simulink model "TCMSSystem"  (R2019b)
settings: configuration reference "ConfigSet_TCMSSystem_Reference" (kept outside this file)
model workspace (MAT data in the model file):
  Prm_TCMSSystem : Simulink.Parameter (value not decoded)
  SampleTime = 0.05
symbols that are objects in the model workspace (value not decoded): Prm_TCMSSystem
undefined symbols (not defined in the file): ADDIntervention, AK1Status, AK2Status, AKContactorStatus, AllDoorsClosed, AllLeftDoorsClosed, AllRightDoorsClosed, APS1Fault, APS1Isolated, APS1OutputVoltage, APS1Status, APS2Fault, APS2Isolated, APS2OutputVoltage, APS2Status, APSKAKContactor, ASCOEnd1, ASCOEnd2, ATBMode, ATCBypassMode, ATCStatusNotOK, ATOMode, ATPLowSpeedCutoutStatus, ATPMode, AuxCompressor, BatteryCurrent, BatteryIsolationContactor, BatteryTemperature, BatteryVoltage, BCG1Fault, BCG1Isolated, BCG1IsolationFailed, BCG1OutputCurrent, BCG1Status, BCG2Fault, BCG2Isolated, BCG2OutputCurrent, BCG2Status, BCGOutputVoltage, BECU1AxleLockedWheelSet1, BECU2AxleLockedWheelSet2, BECUFaulty, BECUMajorFault, BECUMinorFault, BECUStatus, BIC1Inside, BIC1Outside, BIC2Inside, BIC2Outside, Bogie, Bogie1WSPStatus, Bogie2WSPStatus, BogieFaulty, BogieIsolationStatus, BogieSupportedMass, BrakeCylinderPressureGauge, BrakeLoopCBTripped, BrakeLoopOpenTL, BrakeTrainLineStatus, BrakingDemand ... (+215)
libraries: TimersLib x257, simulink x137, LatchesLib x42, VectorOperationsLib x15, TestBenchLib x12, MathOperationsLib x2, FiltersLib x1
(part 15 of 16)

== system TCMSSystem/TCMSSystemPerVehicle/EnabledTCMSVehicle/OutputsPacking/TCMSDisplayOutputs/TCMSMessageEvents/New46EventsMessage/Associated TCMS Fault ID42 ==
  State : Inport
  Bus Creator1 : BusCreator  Inputs=2  OutDataTypeStr=Bus: BD_TCMSSystem_Out_Vehicle_Display_Message  NonVirtualBus=on
  Constant : Constant  Value=MessageID
  Data Type Conversion : DataTypeConversion
  Message : Outport  VectorParamsAs1DForOutWhenUnconnected=off
  wires:
  Data Type Conversion/1 -> Bus Creator1/2  "MessageStatus"
  Constant/1 -> Bus Creator1/1  "MessageID"
  State/1 -> Data Type Conversion/1
  Bus Creator1/1 -> Message/1

== system TCMSSystem/TCMSSystemPerVehicle/EnabledTCMSVehicle/OutputsPacking/TCMSDisplayOutputs/TCMSMessageEvents/New46EventsMessage/Associated TCMS Fault ID43 ==
  State : Inport
  Bus Creator1 : BusCreator  Inputs=2  OutDataTypeStr=Bus: BD_TCMSSystem_Out_Vehicle_Display_Message  NonVirtualBus=on
  Constant : Constant  Value=MessageID
  Data Type Conversion : DataTypeConversion
  Message : Outport  VectorParamsAs1DForOutWhenUnconnected=off
  wires:
  Bus Creator1/1 -> Message/1
  State/1 -> Data Type Conversion/1
  Constant/1 -> Bus Creator1/1  "MessageID"
  Data Type Conversion/1 -> Bus Creator1/2  "MessageStatus"

== system TCMSSystem/TCMSSystemPerVehicle/EnabledTCMSVehicle/OutputsPacking/TCMSDisplayOutputs/TCMSMessageEvents/New46EventsMessage/Associated TCMS Fault ID44 ==
  State : Inport
  Bus Creator1 : BusCreator  Inputs=2  OutDataTypeStr=Bus: BD_TCMSSystem_Out_Vehicle_Display_Message  NonVirtualBus=on
  Constant : Constant  Value=MessageID
  Data Type Conversion : DataTypeConversion
  Message : Outport  VectorParamsAs1DForOutWhenUnconnected=off
  wires:
  Data Type Conversion/1 -> Bus Creator1/2  "MessageStatus"
  Constant/1 -> Bus Creator1/1  "MessageID"
  State/1 -> Data Type Conversion/1
  Bus Creator1/1 -> Message/1

== system TCMSSystem/TCMSSystemPerVehicle/EnabledTCMSVehicle/OutputsPacking/TCMSDisplayOutputs/TCMSMessageEvents/New46EventsMessage/Associated TCMS Fault ID45 ==
  State : Inport
  Bus Creator1 : BusCreator  Inputs=2  OutDataTypeStr=Bus: BD_TCMSSystem_Out_Vehicle_Display_Message  NonVirtualBus=on
  Constant : Constant  Value=MessageID
  Data Type Conversion : DataTypeConversion
  Message : Outport  VectorParamsAs1DForOutWhenUnconnected=off
  wires:
  Data Type Conversion/1 -> Bus Creator1/2  "MessageStatus"
  Constant/1 -> Bus Creator1/1  "MessageID"
  State/1 -> Data Type Conversion/1
  Bus Creator1/1 -> Message/1

== system TCMSSystem/TCMSSystemPerVehicle/EnabledTCMSVehicle/OutputsPacking/TCMSDisplayOutputs/TCMSMessageEvents/New46EventsMessage/Associated TCMS Fault ID46 ==
  State : Inport
  Bus Creator1 : BusCreator  Inputs=2  OutDataTypeStr=Bus: BD_TCMSSystem_Out_Vehicle_Display_Message  NonVirtualBus=on
  Constant : Constant  Value=MessageID
  Data Type Conversion : DataTypeConversion
  Message : Outport  VectorParamsAs1DForOutWhenUnconnected=off
  wires:
  Bus Creator1/1 -> Message/1
  State/1 -> Data Type Conversion/1
  Constant/1 -> Bus Creator1/1  "MessageID"
  Data Type Conversion/1 -> Bus Creator1/2  "MessageStatus"

== system TCMSSystem/TCMSSystemPerVehicle/EnabledTCMSVehicle/OutputsPacking/TCMSDisplayOutputs/TCMSMessageEvents/New46EventsMessage/Associated TCMS Fault ID47 ==
  State : Inport
  Bus Creator1 : BusCreator  Inputs=2  OutDataTypeStr=Bus: BD_TCMSSystem_Out_Vehicle_Display_Message  NonVirtualBus=on
  Constant : Constant  Value=MessageID
  Data Type Conversion : DataTypeConversion
  Message : Outport  VectorParamsAs1DForOutWhenUnconnected=off
  wires:
  Data Type Conversion/1 -> Bus Creator1/2  "MessageStatus"
  Constant/1 -> Bus Creator1/1  "MessageID"
  State/1 -> Data Type Conversion/1
  Bus Creator1/1 -> Message/1

== system TCMSSystem/TCMSSystemPerVehicle/EnabledTCMSVehicle/OutputsPacking/TCMSDisplayOutputs/TCMSMessageEvents/New46EventsMessage/Associated TCMS Fault ID48 ==
  State : Inport
  Bus Creator1 : BusCreator  Inputs=2  OutDataTypeStr=Bus: BD_TCMSSystem_Out_Vehicle_Display_Message  NonVirtualBus=on
  Constant : Constant  Value=MessageID
  Data Type Conversion : DataTypeConversion
  Message : Outport  VectorParamsAs1DForOutWhenUnconnected=off
  wires:
  Bus Creator1/1 -> Message/1
  State/1 -> Data Type Conversion/1
  Constant/1 -> Bus Creator1/1  "MessageID"
  Data Type Conversion/1 -> Bus Creator1/2  "MessageStatus"

== system TCMSSystem/TCMSSystemPerVehicle/EnabledTCMSVehicle/OutputsPacking/TCMSDisplayOutputs/TCMSMessageEvents/New46EventsMessage/Associated TCMS Fault ID50 ==
  State : Inport
  Bus Creator1 : BusCreator  Inputs=2  OutDataTypeStr=Bus: BD_TCMSSystem_Out_Vehicle_Display_Message  NonVirtualBus=on
  Constant : Constant  Value=MessageID
  Data Type Conversion : DataTypeConversion
  Message : Outport  VectorParamsAs1DForOutWhenUnconnected=off
  wires:
  Bus Creator1/1 -> Message/1
  State/1 -> Data Type Conversion/1
  Constant/1 -> Bus Creator1/1  "MessageID"
  Data Type Conversion/1 -> Bus Creator1/2  "MessageStatus"

== system TCMSSystem/TCMSSystemPerVehicle/EnabledTCMSVehicle/OutputsPacking/TCMSDisplayOutputs/TCMSMessageEvents/New46EventsMessage/Associated TCMS Fault ID53 ==
  State : Inport
  Bus Creator1 : BusCreator  Inputs=2  OutDataTypeStr=Bus: BD_TCMSSystem_Out_Vehicle_Display_Message  NonVirtualBus=on
  Constant : Constant  Value=MessageID
  Data Type Conversion : DataTypeConversion
  Message : Outport  VectorParamsAs1DForOutWhenUnconnected=off
  wires:
  Bus Creator1/1 -> Message/1
  State/1 -> Data Type Conversion/1
  Constant/1 -> Bus Creator1/1  "MessageID"
  Data Type Conversion/1 -> Bus Creator1/2  "MessageStatus"

== system TCMSSystem/TCMSSystemPerVehicle/EnabledTCMSVehicle/OutputsPacking/TCMSDisplayOutputs/TCMSMessageEvents/New46EventsMessage/Associated TCMS Fault ID54 ==
  State : Inport
  Bus Creator1 : BusCreator  Inputs=2  OutDataTypeStr=Bus: BD_TCMSSystem_Out_Vehicle_Display_Message  NonVirtualBus=on
  Constant : Constant  Value=MessageID
  Data Type Conversion : DataTypeConversion
  Message : Outport  VectorParamsAs1DForOutWhenUnconnected=off
  wires:
  Data Type Conversion/1 -> Bus Creator1/2  "MessageStatus"
  Constant/1 -> Bus Creator1/1  "MessageID"
  State/1 -> Data Type Conversion/1
  Bus Creator1/1 -> Message/1

== system TCMSSystem/TCMSSystemPerVehicle/EnabledTCMSVehicle/OutputsPacking/TCMSDisplayOutputs/TCMSMessageEvents/New46EventsMessage/Associated TCMS Fault ID55 ==
  State : Inport
  Bus Creator1 : BusCreator  Inputs=2  OutDataTypeStr=Bus: BD_TCMSSystem_Out_Vehicle_Display_Message  NonVirtualBus=on
  Constant : Constant  Value=MessageID
  Data Type Conversion : DataTypeConversion
  Message : Outport  VectorParamsAs1DForOutWhenUnconnected=off
  wires:
  Bus Creator1/1 -> Message/1
  State/1 -> Data Type Conversion/1
  Constant/1 -> Bus Creator1/1  "MessageID"
  Data Type Conversion/1 -> Bus Creator1/2  "MessageStatus"

== system TCMSSystem/TCMSSystemPerVehicle/EnabledTCMSVehicle/OutputsPacking/TCMSDisplayOutputs/TCMSMessageEvents/New46EventsMessage/Associated TCMS Fault ID56 ==
  State : Inport
  Bus Creator1 : BusCreator  Inputs=2  OutDataTypeStr=Bus: BD_TCMSSystem_Out_Vehicle_Display_Message  NonVirtualBus=on
  Constant : Constant  Value=MessageID
  Data Type Conversion : DataTypeConversion
  Message : Outport  VectorParamsAs1DForOutWhenUnconnected=off
  wires:
  Data Type Conversion/1 -> Bus Creator1/2  "MessageStatus"
  Constant/1 -> Bus Creator1/1  "MessageID"
  State/1 -> Data Type Conversion/1
  Bus Creator1/1 -> Message/1

== system TCMSSystem/TCMSSystemPerVehicle/EnabledTCMSVehicle/OutputsPacking/TCMSDisplayOutputs/TCMSMessageEvents/New46EventsMessage/Associated TCMS Fault ID57 ==
  State : Inport
  Bus Creator1 : BusCreator  Inputs=2  OutDataTypeStr=Bus: BD_TCMSSystem_Out_Vehicle_Display_Message  NonVirtualBus=on
  Constant : Constant  Value=MessageID
  Data Type Conversion : DataTypeConversion
  Message : Outport  VectorParamsAs1DForOutWhenUnconnected=off
  wires:
  Bus Creator1/1 -> Message/1
  State/1 -> Data Type Conversion/1
  Constant/1 -> Bus Creator1/1  "MessageID"
  Data Type Conversion/1 -> Bus Creator1/2  "MessageStatus"

== system TCMSSystem/TCMSSystemPerVehicle/EnabledTCMSVehicle/OutputsPacking/TCMSDisplayOutputs/TCMSMessageEvents/New46EventsMessage/Associated TCMS Fault ID6 ==
  State : Inport
  Bus Creator1 : BusCreator  Inputs=2  OutDataTypeStr=Bus: BD_TCMSSystem_Out_Vehicle_Display_Message  NonVirtualBus=on
  Constant : Constant  Value=MessageID
  Data Type Conversion : DataTypeConversion
  Message : Outport  VectorParamsAs1DForOutWhenUnconnected=off
  wires:
  Bus Creator1/1 -> Message/1
  State/1 -> Data Type Conversion/1
  Constant/1 -> Bus Creator1/1  "MessageID"
  Data Type Conversion/1 -> Bus Creator1/2  "MessageStatus"

== system TCMSSystem/TCMSSystemPerVehicle/EnabledTCMSVehicle/OutputsPacking/TCMSDisplayOutputs/TCMSMessageEvents/New46EventsMessage/Associated TCMS Fault ID7 ==
  State : Inport
  Bus Creator1 : BusCreator  Inputs=2  OutDataTypeStr=Bus: BD_TCMSSystem_Out_Vehicle_Display_Message  NonVirtualBus=on
  Constant : Constant  Value=MessageID
  Data Type Conversion : DataTypeConversion
  Message : Outport  VectorParamsAs1DForOutWhenUnconnected=off
  wires:
  Data Type Conversion/1 -> Bus Creator1/2  "MessageStatus"
  Constant/1 -> Bus Creator1/1  "MessageID"
  State/1 -> Data Type Conversion/1
  Bus Creator1/1 -> Message/1

== system TCMSSystem/TCMSSystemPerVehicle/EnabledTCMSVehicle/OutputsPacking/TCMSDisplayOutputs/TCMSMessageEvents/New46EventsMessage/Associated TCMS Fault ID8 ==
  State : Inport
  Bus Creator1 : BusCreator  Inputs=2  OutDataTypeStr=Bus: BD_TCMSSystem_Out_Vehicle_Display_Message  NonVirtualBus=on
  Constant : Constant  Value=MessageID
  Data Type Conversion : DataTypeConversion
  Message : Outport  VectorParamsAs1DForOutWhenUnconnected=off
  wires:
  Bus Creator1/1 -> Message/1
  State/1 -> Data Type Conversion/1
  Constant/1 -> Bus Creator1/1  "MessageID"
  Data Type Conversion/1 -> Bus Creator1/2  "MessageStatus"

== system TCMSSystem/TCMSSystemPerVehicle/EnabledTCMSVehicle/OutputsPacking/TCMSDisplayOutputs/TCMSMessageEvents/PantographSystemFaults/Associated TCMS Fault ID24 ==
  State : Inport
  Bus Creator1 : BusCreator  Inputs=2  OutDataTypeStr=Bus: BD_TCMSSystem_Out_Vehicle_Display_Message  NonVirtualBus=on
  Constant : Constant  Value=MessageID
  Data Type Conversion : DataTypeConversion
  Message : Outport  VectorParamsAs1DForOutWhenUnconnected=off
  wires:
  Bus Creator1/1 -> Message/1
  State/1 -> Data Type Conversion/1
  Constant/1 -> Bus Creator1/1  "MessageID"
  Data Type Conversion/1 -> Bus Creator1/2  "MessageStatus"

== system TCMSSystem/TCMSSystemPerVehicle/EnabledTCMSVehicle/OutputsPacking/TCMSDisplayOutputs/TCMSMessageEvents/PantographSystemFaults/Associated TCMS Fault ID25 ==
  State : Inport
  Bus Creator1 : BusCreator  Inputs=2  OutDataTypeStr=Bus: BD_TCMSSystem_Out_Vehicle_Display_Message  NonVirtualBus=on
  Constant : Constant  Value=MessageID
  Data Type Conversion : DataTypeConversion
  Message : Outport  VectorParamsAs1DForOutWhenUnconnected=off
  wires:
  Data Type Conversion/1 -> Bus Creator1/2  "MessageStatus"
  Constant/1 -> Bus Creator1/1  "MessageID"
  State/1 -> Data Type Conversion/1
  Bus Creator1/1 -> Message/1

== system TCMSSystem/TCMSSystemPerVehicle/EnabledTCMSVehicle/OutputsPacking/TCMSDisplayOutputs/TCMSMessageEvents/PantographSystemFaults/Associated TCMS Fault ID26 ==
  State : Inport
  Bus Creator1 : BusCreator  Inputs=2  OutDataTypeStr=Bus: BD_TCMSSystem_Out_Vehicle_Display_Message  NonVirtualBus=on
  Constant : Constant  Value=MessageID
  Data Type Conversion : DataTypeConversion
  Message : Outport  VectorParamsAs1DForOutWhenUnconnected=off
  wires:
  Bus Creator1/1 -> Message/1
  State/1 -> Data Type Conversion/1
  Constant/1 -> Bus Creator1/1  "MessageID"
  Data Type Conversion/1 -> Bus Creator1/2  "MessageStatus"

== system TCMSSystem/TCMSSystemPerVehicle/EnabledTCMSVehicle/OutputsPacking/TCMSDisplayOutputs/TCMSMessageEvents/TCMSSystemFaults/Associated TCMS Fault ID1 ==
  State : Inport
  Bus Creator1 : BusCreator  Inputs=2  OutDataTypeStr=Bus: BD_TCMSSystem_Out_Vehicle_Display_Message  NonVirtualBus=on
  Constant : Constant  Value=MessageID
  Data Type Conversion : DataTypeConversion
  Message : Outport  VectorParamsAs1DForOutWhenUnconnected=off
  wires:
  Data Type Conversion/1 -> Bus Creator1/2  "MessageStatus"
  Constant/1 -> Bus Creator1/1  "MessageID"
  State/1 -> Data Type Conversion/1
  Bus Creator1/1 -> Message/1

== system TCMSSystem/TCMSSystemPerVehicle/EnabledTCMSVehicle/OutputsPacking/TCMSDisplayOutputs/TCMSMessageEvents/TCMSSystemFaults/Associated TCMS Fault ID100 ==
  State : Inport
  Bus Creator1 : BusCreator  Inputs=2  OutDataTypeStr=Bus: BD_TCMSSystem_Out_Vehicle_Display_Message  NonVirtualBus=on
  Constant : Constant  Value=MessageID
  Data Type Conversion : DataTypeConversion
  Message : Outport  VectorParamsAs1DForOutWhenUnconnected=off
  wires:
  Data Type Conversion/1 -> Bus Creator1/2  "MessageStatus"
  Constant/1 -> Bus Creator1/1  "MessageID"
  State/1 -> Data Type Conversion/1
  Bus Creator1/1 -> Message/1

== system TCMSSystem/TCMSSystemPerVehicle/EnabledTCMSVehicle/OutputsPacking/TCMSDisplayOutputs/TCMSMessageEvents/TCMSSystemFaults/Associated TCMS Fault ID101 ==
  State : Inport
  Bus Creator1 : BusCreator  Inputs=2  OutDataTypeStr=Bus: BD_TCMSSystem_Out_Vehicle_Display_Message  NonVirtualBus=on
  Constant : Constant  Value=MessageID
  Data Type Conversion : DataTypeConversion
  Message : Outport  VectorParamsAs1DForOutWhenUnconnected=off
  wires:
  Bus Creator1/1 -> Message/1
  State/1 -> Data Type Conversion/1
  Constant/1 -> Bus Creator1/1  "MessageID"
  Data Type Conversion/1 -> Bus Creator1/2  "MessageStatus"

== system TCMSSystem/TCMSSystemPerVehicle/EnabledTCMSVehicle/OutputsPacking/TCMSDisplayOutputs/TCMSMessageEvents/TCMSSystemFaults/Associated TCMS Fault ID21 ==
  State : Inport
  Bus Creator1 : BusCreator  Inputs=2  OutDataTypeStr=Bus: BD_TCMSSystem_Out_Vehicle_Display_Message  NonVirtualBus=on
  Constant : Constant  Value=MessageID
  Data Type Conversion : DataTypeConversion
  Message : Outport  VectorParamsAs1DForOutWhenUnconnected=off
  wires:
  Bus Creator1/1 -> Message/1
  State/1 -> Data Type Conversion/1
  Constant/1 -> Bus Creator1/1  "MessageID"
  Data Type Conversion/1 -> Bus Creator1/2  "MessageStatus"

== system TCMSSystem/TCMSSystemPerVehicle/EnabledTCMSVehicle/OutputsPacking/TCMSDisplayOutputs/TCMSMessageEvents/TCMSSystemFaults/Associated TCMS Fault ID97 ==
  State : Inport
  Bus Creator1 : BusCreator  Inputs=2  OutDataTypeStr=Bus: BD_TCMSSystem_Out_Vehicle_Display_Message  NonVirtualBus=on
  Constant : Constant  Value=MessageID
  Data Type Conversion : DataTypeConversion
  Message : Outport  VectorParamsAs1DForOutWhenUnconnected=off
  wires:
  Bus Creator1/1 -> Message/1
  State/1 -> Data Type Conversion/1
  Constant/1 -> Bus Creator1/1  "MessageID"
  Data Type Conversion/1 -> Bus Creator1/2  "MessageStatus"

== system TCMSSystem/TCMSSystemPerVehicle/EnabledTCMSVehicle/OutputsPacking/TCMSDisplayOutputs/TCMSMessageEvents/TCMSSystemFaults/Associated TCMS Fault ID98 ==
  State : Inport
  Bus Creator1 : BusCreator  Inputs=2  OutDataTypeStr=Bus: BD_TCMSSystem_Out_Vehicle_Display_Message  NonVirtualBus=on
  Constant : Constant  Value=MessageID
  Data Type Conversion : DataTypeConversion
  Message : Outport  VectorParamsAs1DForOutWhenUnconnected=off
  wires:
  Data Type Conversion/1 -> Bus Creator1/2  "MessageStatus"
  Constant/1 -> Bus Creator1/1  "MessageID"
  State/1 -> Data Type Conversion/1
  Bus Creator1/1 -> Message/1

== system TCMSSystem/TCMSSystemPerVehicle/EnabledTCMSVehicle/OutputsPacking/TCMSDisplayOutputs/TCMSMessageEvents/TCMSSystemFaults/Associated TCMS Fault ID99 ==
  State : Inport
  Bus Creator1 : BusCreator  Inputs=2  OutDataTypeStr=Bus: BD_TCMSSystem_Out_Vehicle_Display_Message  NonVirtualBus=on
  Constant : Constant  Value=MessageID
  Data Type Conversion : DataTypeConversion
  Message : Outport  VectorParamsAs1DForOutWhenUnconnected=off
  wires:
  Bus Creator1/1 -> Message/1
  State/1 -> Data Type Conversion/1
  Constant/1 -> Bus Creator1/1  "MessageID"
  Data Type Conversion/1 -> Bus Creator1/2  "MessageStatus"

== system TCMSSystem/TCMSSystemPerVehicle/EnabledTCMSVehicle/OutputsPacking/TCMSDisplayOutputs/TCMSMessageEvents/TractionSystemFaults/Associated TCMS Fault ID1 ==
  State : Inport
  Bus Creator1 : BusCreator  Inputs=2  OutDataTypeStr=Bus: BD_TCMSSystem_Out_Vehicle_Display_Message  NonVirtualBus=on
  Constant : Constant  Value=MessageID
  Data Type Conversion : DataTypeConversion
  Message : Outport  VectorParamsAs1DForOutWhenUnconnected=off
  wires:
  Data Type Conversion/1 -> Bus Creator1/2  "MessageStatus"
  Constant/1 -> Bus Creator1/1  "MessageID"
  State/1 -> Data Type Conversion/1
  Bus Creator1/1 -> Message/1

== system TCMSSystem/TCMSSystemPerVehicle/EnabledTCMSVehicle/OutputsPacking/TCMSDisplayOutputs/TCMSMessageEvents/TractionSystemFaults/Associated TCMS Fault ID34 ==
  State : Inport
  Bus Creator1 : BusCreator  Inputs=2  OutDataTypeStr=Bus: BD_TCMSSystem_Out_Vehicle_Display_Message  NonVirtualBus=on
  Constant : Constant  Value=MessageID
  Data Type Conversion : DataTypeConversion
  Message : Outport  VectorParamsAs1DForOutWhenUnconnected=off
  wires:
  Data Type Conversion/1 -> Bus Creator1/2  "MessageStatus"
  Constant/1 -> Bus Creator1/1  "MessageID"
  State/1 -> Data Type Conversion/1
  Bus Creator1/1 -> Message/1

== system TCMSSystem/TCMSSystemPerVehicle/EnabledTCMSVehicle/OutputsPacking/TCMSDisplayOutputs/TCMSMessageEvents/TractionSystemFaults/Associated TCMS Fault ID35 ==
  State : Inport
  Bus Creator1 : BusCreator  Inputs=2  OutDataTypeStr=Bus: BD_TCMSSystem_Out_Vehicle_Display_Message  NonVirtualBus=on
  Constant : Constant  Value=MessageID
  Data Type Conversion : DataTypeConversion
  Message : Outport  VectorParamsAs1DForOutWhenUnconnected=off
  wires:
  Bus Creator1/1 -> Message/1
  State/1 -> Data Type Conversion/1
  Constant/1 -> Bus Creator1/1  "MessageID"
  Data Type Conversion/1 -> Bus Creator1/2  "MessageStatus"

== system TCMSSystem/TCMSSystemPerVehicle/EnabledTCMSVehicle/OutputsPacking/TCMSDisplayOutputs/TCMSMessageEvents/TractionSystemFaults/Associated TCMS Fault ID36 ==
  State : Inport
  Bus Creator1 : BusCreator  Inputs=2  OutDataTypeStr=Bus: BD_TCMSSystem_Out_Vehicle_Display_Message  NonVirtualBus=on
  Constant : Constant  Value=MessageID
  Data Type Conversion : DataTypeConversion
  Message : Outport  VectorParamsAs1DForOutWhenUnconnected=off
  wires:
  Data Type Conversion/1 -> Bus Creator1/2  "MessageStatus"
  Constant/1 -> Bus Creator1/1  "MessageID"
  State/1 -> Data Type Conversion/1
  Bus Creator1/1 -> Message/1

== system TCMSSystem/TCMSSystemPerVehicle/EnabledTCMSVehicle/OutputsPacking/TCMSDisplayOutputs/TCMSMessageEvents/TractionSystemFaults/Associated TCMS Fault ID37 ==
  State : Inport
  Bus Creator1 : BusCreator  Inputs=2  OutDataTypeStr=Bus: BD_TCMSSystem_Out_Vehicle_Display_Message  NonVirtualBus=on
  Constant : Constant  Value=MessageID
  Data Type Conversion : DataTypeConversion
  Message : Outport  VectorParamsAs1DForOutWhenUnconnected=off
  wires:
  Bus Creator1/1 -> Message/1
  State/1 -> Data Type Conversion/1
  Constant/1 -> Bus Creator1/1  "MessageID"
  Data Type Conversion/1 -> Bus Creator1/2  "MessageStatus"

== system TCMSSystem/TCMSSystemPerVehicle/EnabledTCMSVehicle/OutputsPacking/TCMSDisplayOutputs/TCMSMessageEvents/TractionSystemFaults/Associated TCMS Fault ID38 ==
  State : Inport
  Bus Creator1 : BusCreator  Inputs=2  OutDataTypeStr=Bus: BD_TCMSSystem_Out_Vehicle_Display_Message  NonVirtualBus=on
  Constant : Constant  Value=MessageID
  Data Type Conversion : DataTypeConversion
  Message : Outport  VectorParamsAs1DForOutWhenUnconnected=off
  wires:
  Data Type Conversion/1 -> Bus Creator1/2  "MessageStatus"
  Constant/1 -> Bus Creator1/1  "MessageID"
  State/1 -> Data Type Conversion/1
  Bus Creator1/1 -> Message/1

== system TCMSSystem/TCMSSystemPerVehicle/EnabledTCMSVehicle/OutputsPacking/TCMSDisplayOutputs/TCMSMessageEvents/TractionSystemFaults/Associated TCMS Fault ID39 ==
  State : Inport
  Bus Creator1 : BusCreator  Inputs=2  OutDataTypeStr=Bus: BD_TCMSSystem_Out_Vehicle_Display_Message  NonVirtualBus=on
  Constant : Constant  Value=MessageID
  Data Type Conversion : DataTypeConversion
  Message : Outport  VectorParamsAs1DForOutWhenUnconnected=off
  wires:
  Bus Creator1/1 -> Message/1
  State/1 -> Data Type Conversion/1
  Constant/1 -> Bus Creator1/1  "MessageID"
  Data Type Conversion/1 -> Bus Creator1/2  "MessageStatus"

== system TCMSSystem/TCMSSystemPerVehicle/EnabledTCMSVehicle/OutputsPacking/TCMSDisplayOutputs/TCMSMessageEvents/TractionSystemFaults/Associated TCMS Fault ID40 ==
  State : Inport
  Bus Creator1 : BusCreator  Inputs=2  OutDataTypeStr=Bus: BD_TCMSSystem_Out_Vehicle_Display_Message  NonVirtualBus=on
  Constant : Constant  Value=MessageID
  Data Type Conversion : DataTypeConversion
  Message : Outport  VectorParamsAs1DForOutWhenUnconnected=off
  wires:
  Bus Creator1/1 -> Message/1
  State/1 -> Data Type Conversion/1
  Constant/1 -> Bus Creator1/1  "MessageID"
  Data Type Conversion/1 -> Bus Creator1/2  "MessageStatus"

== system TCMSSystem/TCMSSystemPerVehicle/EnabledTCMSVehicle/OutputsPacking/TCMSDisplayOutputs/TCMSMessageEvents/TractionSystemFaults/Associated TCMS Fault ID41 ==
  State : Inport
  Bus Creator1 : BusCreator  Inputs=2  OutDataTypeStr=Bus: BD_TCMSSystem_Out_Vehicle_Display_Message  NonVirtualBus=on
  Constant : Constant  Value=MessageID
  Data Type Conversion : DataTypeConversion
  Message : Outport  VectorParamsAs1DForOutWhenUnconnected=off
  wires:
  Data Type Conversion/1 -> Bus Creator1/2  "MessageStatus"
  Constant/1 -> Bus Creator1/1  "MessageID"
  State/1 -> Data Type Conversion/1
  Bus Creator1/1 -> Message/1

== system TCMSSystem/TCMSSystemPerVehicle/EnabledTCMSVehicle/OutputsPacking/TCMSDisplayOutputs/TCMSMessageEvents/TractionSystemFaults/Associated TCMS Fault ID42 ==
  State : Inport
  Bus Creator1 : BusCreator  Inputs=2  OutDataTypeStr=Bus: BD_TCMSSystem_Out_Vehicle_Display_Message  NonVirtualBus=on
  Constant : Constant  Value=MessageID
  Data Type Conversion : DataTypeConversion
  Message : Outport  VectorParamsAs1DForOutWhenUnconnected=off
  wires:
  Bus Creator1/1 -> Message/1
  State/1 -> Data Type Conversion/1
  Constant/1 -> Bus Creator1/1  "MessageID"
  Data Type Conversion/1 -> Bus Creator1/2  "MessageStatus"

== system TCMSSystem/TCMSSystemPerVehicle/EnabledTCMSVehicle/OutputsPacking/TCMSDisplayOutputs/TCMSMessageEvents/TractionSystemFaults/Associated TCMS Fault ID43 ==
  State : Inport
  Bus Creator1 : BusCreator  Inputs=2  OutDataTypeStr=Bus: BD_TCMSSystem_Out_Vehicle_Display_Message  NonVirtualBus=on
  Constant : Constant  Value=MessageID
  Data Type Conversion : DataTypeConversion
  Message : Outport  VectorParamsAs1DForOutWhenUnconnected=off
  wires:
  Data Type Conversion/1 -> Bus Creator1/2  "MessageStatus"
  Constant/1 -> Bus Creator1/1  "MessageID"
  State/1 -> Data Type Conversion/1
  Bus Creator1/1 -> Message/1

== system TCMSSystem/TCMSSystemPerVehicle/EnabledTCMSVehicle/OutputsPacking/TCMSDisplayOutputs/TCMSMessageEvents/TractionSystemFaults/Associated TCMS Fault ID44 ==
  State : Inport
  Bus Creator1 : BusCreator  Inputs=2  OutDataTypeStr=Bus: BD_TCMSSystem_Out_Vehicle_Display_Message  NonVirtualBus=on
  Constant : Constant  Value=MessageID
  Data Type Conversion : DataTypeConversion
  Message : Outport  VectorParamsAs1DForOutWhenUnconnected=off
  wires:
  Bus Creator1/1 -> Message/1
  State/1 -> Data Type Conversion/1
  Constant/1 -> Bus Creator1/1  "MessageID"
  Data Type Conversion/1 -> Bus Creator1/2  "MessageStatus"

== system TCMSSystem/TCMSSystemPerVehicle/EnabledTCMSVehicle/OutputsPacking/TCMSDisplayOutputs/TCMSMessageEvents/TractionSystemFaults/Associated TCMS Fault ID45 ==
  State : Inport
  Bus Creator1 : BusCreator  Inputs=2  OutDataTypeStr=Bus: BD_TCMSSystem_Out_Vehicle_Display_Message  NonVirtualBus=on
  Constant : Constant  Value=MessageID
  Data Type Conversion : DataTypeConversion
  Message : Outport  VectorParamsAs1DForOutWhenUnconnected=off
  wires:
  Data Type Conversion/1 -> Bus Creator1/2  "MessageStatus"
  Constant/1 -> Bus Creator1/1  "MessageID"
  State/1 -> Data Type Conversion/1
  Bus Creator1/1 -> Message/1

== system TCMSSystem/TCMSSystemPerVehicle/EnabledTCMSVehicle/OutputsPacking/TCMSDisplayOutputs/TCMSMessageEvents/TractionSystemFaults/Associated TCMS Fault ID46 ==
  State : Inport
  Bus Creator1 : BusCreator  Inputs=2  OutDataTypeStr=Bus: BD_TCMSSystem_Out_Vehicle_Display_Message  NonVirtualBus=on
  Constant : Constant  Value=MessageID
  Data Type Conversion : DataTypeConversion
  Message : Outport  VectorParamsAs1DForOutWhenUnconnected=off
  wires:
  Bus Creator1/1 -> Message/1
  State/1 -> Data Type Conversion/1
  Constant/1 -> Bus Creator1/1  "MessageID"
  Data Type Conversion/1 -> Bus Creator1/2  "MessageStatus"

== system TCMSSystem/TCMSSystemPerVehicle/EnabledTCMSVehicle/OutputsPacking/TCMSDisplayOutputs/TCMSMessageEvents/TractionSystemFaults/Associated TCMS Fault ID47 ==
  State : Inport
  Bus Creator1 : BusCreator  Inputs=2  OutDataTypeStr=Bus: BD_TCMSSystem_Out_Vehicle_Display_Message  NonVirtualBus=on
  Constant : Constant  Value=MessageID
  Data Type Conversion : DataTypeConversion
  Message : Outport  VectorParamsAs1DForOutWhenUnconnected=off
  wires:
  Data Type Conversion/1 -> Bus Creator1/2  "MessageStatus"
  Constant/1 -> Bus Creator1/1  "MessageID"
  State/1 -> Data Type Conversion/1
  Bus Creator1/1 -> Message/1

== system TCMSSystem/TCMSSystemPerVehicle/EnabledTCMSVehicle/OutputsPacking/TCMSDisplayOutputs/TCMSMessageEvents/TractionSystemFaults/Associated TCMS Fault ID48 ==
  State : Inport
  Bus Creator1 : BusCreator  Inputs=2  OutDataTypeStr=Bus: BD_TCMSSystem_Out_Vehicle_Display_Message  NonVirtualBus=on
  Constant : Constant  Value=MessageID
  Data Type Conversion : DataTypeConversion
  Message : Outport  VectorParamsAs1DForOutWhenUnconnected=off
  wires:
  Bus Creator1/1 -> Message/1
  State/1 -> Data Type Conversion/1
  Constant/1 -> Bus Creator1/1  "MessageID"
  Data Type Conversion/1 -> Bus Creator1/2  "MessageStatus"

== system TCMSSystem/TCMSSystemPerVehicle/EnabledTCMSVehicle/OutputsPacking/TCMSDisplayOutputs/TCMSMessageEvents/TractionSystemFaults/Associated TCMS Fault ID49 ==
  State : Inport
  Bus Creator1 : BusCreator  Inputs=2  OutDataTypeStr=Bus: BD_TCMSSystem_Out_Vehicle_Display_Message  NonVirtualBus=on
  Constant : Constant  Value=MessageID
  Data Type Conversion : DataTypeConversion
  Message : Outport  VectorParamsAs1DForOutWhenUnconnected=off
  wires:
  Data Type Conversion/1 -> Bus Creator1/2  "MessageStatus"
  Constant/1 -> Bus Creator1/1  "MessageID"
  State/1 -> Data Type Conversion/1
  Bus Creator1/1 -> Message/1

== system TCMSSystem/TCMSSystemPerVehicle/EnabledTCMSVehicle/OutputsPacking/TCMSDisplayOutputs/TCMSMessageEvents/TractionSystemFaults/Associated TCMS Fault ID50 ==
  State : Inport
  Bus Creator1 : BusCreator  Inputs=2  OutDataTypeStr=Bus: BD_TCMSSystem_Out_Vehicle_Display_Message  NonVirtualBus=on
  Constant : Constant  Value=MessageID
  Data Type Conversion : DataTypeConversion
  Message : Outport  VectorParamsAs1DForOutWhenUnconnected=off
  wires:
  Bus Creator1/1 -> Message/1
  State/1 -> Data Type Conversion/1
  Constant/1 -> Bus Creator1/1  "MessageID"
  Data Type Conversion/1 -> Bus Creator1/2  "MessageStatus"

== system TCMSSystem/TCMSSystemPerVehicle/EnabledTCMSVehicle/OutputsPacking/TCMSDisplayOutputs/TCMSMessageEvents/TractionSystemFaults/Associated TCMS Fault ID51 ==
  State : Inport
  Bus Creator1 : BusCreator  Inputs=2  OutDataTypeStr=Bus: BD_TCMSSystem_Out_Vehicle_Display_Message  NonVirtualBus=on
  Constant : Constant  Value=MessageID
  Data Type Conversion : DataTypeConversion
  Message : Outport  VectorParamsAs1DForOutWhenUnconnected=off
  wires:
  Data Type Conversion/1 -> Bus Creator1/2  "MessageStatus"
  Constant/1 -> Bus Creator1/1  "MessageID"
  State/1 -> Data Type Conversion/1
  Bus Creator1/1 -> Message/1

== system TCMSSystem/TCMSSystemPerVehicle/EnabledTCMSVehicle/OutputsPacking/TCMSDisplayOutputs/TCMSMessageEvents/TractionSystemFaults/Associated TCMS Fault ID52 ==
  State : Inport
  Bus Creator1 : BusCreator  Inputs=2  OutDataTypeStr=Bus: BD_TCMSSystem_Out_Vehicle_Display_Message  NonVirtualBus=on
  Constant : Constant  Value=MessageID
  Data Type Conversion : DataTypeConversion
  Message : Outport  VectorParamsAs1DForOutWhenUnconnected=off
  wires:
  Data Type Conversion/1 -> Bus Creator1/2  "MessageStatus"
  Constant/1 -> Bus Creator1/1  "MessageID"
  State/1 -> Data Type Conversion/1
  Bus Creator1/1 -> Message/1

== system TCMSSystem/TCMSSystemPerVehicle/EnabledTCMSVehicle/OutputsPacking/TCMSDisplayOutputs/TCMSMessageEvents/TractionSystemFaults/Associated TCMS Fault ID53 ==
  State : Inport
  Bus Creator1 : BusCreator  Inputs=2  OutDataTypeStr=Bus: BD_TCMSSystem_Out_Vehicle_Display_Message  NonVirtualBus=on
  Constant : Constant  Value=MessageID
  Data Type Conversion : DataTypeConversion
  Message : Outport  VectorParamsAs1DForOutWhenUnconnected=off
  wires:
  Bus Creator1/1 -> Message/1
  State/1 -> Data Type Conversion/1
  Constant/1 -> Bus Creator1/1  "MessageID"
  Data Type Conversion/1 -> Bus Creator1/2  "MessageStatus"

== system TCMSSystem/TCMSSystemPerVehicle/EnabledTCMSVehicle/OutputsPacking/TCMSDisplayOutputs/TCMSMessageEvents/TractionSystemFaults/Associated TCMS Fault ID54 ==
  State : Inport
  Bus Creator1 : BusCreator  Inputs=2  OutDataTypeStr=Bus: BD_TCMSSystem_Out_Vehicle_Display_Message  NonVirtualBus=on
  Constant : Constant  Value=MessageID
  Data Type Conversion : DataTypeConversion
  Message : Outport  VectorParamsAs1DForOutWhenUnconnected=off
  wires:
  Data Type Conversion/1 -> Bus Creator1/2  "MessageStatus"
  Constant/1 -> Bus Creator1/1  "MessageID"
  State/1 -> Data Type Conversion/1
  Bus Creator1/1 -> Message/1

== system TCMSSystem/TCMSSystemPerVehicle/EnabledTCMSVehicle/OutputsPacking/TCMSDisplayOutputs/TCMSMessageEvents/TractionSystemFaults/Associated TCMS Fault ID57 ==
  State : Inport
  Bus Creator1 : BusCreator  Inputs=2  OutDataTypeStr=Bus: BD_TCMSSystem_Out_Vehicle_Display_Message  NonVirtualBus=on
  Constant : Constant  Value=MessageID
  Data Type Conversion : DataTypeConversion
  Message : Outport  VectorParamsAs1DForOutWhenUnconnected=off
  wires:
  Bus Creator1/1 -> Message/1
  State/1 -> Data Type Conversion/1
  Constant/1 -> Bus Creator1/1  "MessageID"
  Data Type Conversion/1 -> Bus Creator1/2  "MessageStatus"

== system TCMSSystem/TCMSSystemPerVehicle/EnabledTCMSVehicle/TCMSDoors/DoorsDisplay/TCMSVehicleInfo/Subsystem1/For Each Subsystem1 ==
  Source1 : Inport  Partition=on  PartitionDimension=1  PartitionWidth=1  PartitionOffset=0
  Source2 : Inport  Port=2  Partition=on  PartitionDimension=1  PartitionWidth=1  PartitionOffset=0
  Orientation : Inport  Port=3
  For Each : ForEach  DisableCoverage=on
  Orientation Swap : VectorOperationsLib/Orientation Swap
      settings: SourceProductName=Sydac Utilities
  WireState1 : Outport  ConcatenationDimension=1
  WireState2 : Outport  Port=2  ConcatenationDimension=1
  wires:
  Orientation/1 -> Orientation Swap/3
  Source2/1 -> Orientation Swap/2
  Orientation Swap/2 -> WireState2/1
  Orientation Swap/1 -> WireState1/1
  Source1/1 -> Orientation Swap/1

== system TCMSSystem/TCMSSystemPerVehicle/EnabledTCMSVehicle/TCMSDoors/DoorsDisplay/TCMSVehicleInfo/Subsystem1/For Each Subsystem2 ==
  Source1 : Inport  Partition=on  PartitionDimension=1  PartitionWidth=1  PartitionOffset=0
  Source2 : Inport  Port=2  Partition=on  PartitionDimension=1  PartitionWidth=1  PartitionOffset=0
  Orientation : Inport  Port=3
  For Each : ForEach  DisableCoverage=on
  Orientation Swap : VectorOperationsLib/Orientation Swap
      settings: SourceProductName=Sydac Utilities
  WireState1 : Outport  ConcatenationDimension=1
  WireState2 : Outport  Port=2  ConcatenationDimension=1
  wires:
  Source1/1 -> Orientation Swap/1
  Orientation Swap/1 -> WireState1/1
  Orientation Swap/2 -> WireState2/1
  Source2/1 -> Orientation Swap/2
  Orientation/1 -> Orientation Swap/3

== system TCMSSystem/TCMSSystemPerVehicle/EnabledTCMSVehicle/TCMSDoors/DoorsDisplay/TCMSVehicleInfo/Subsystem1/For Each Subsystem3 ==
  Source1 : Inport  Partition=on  PartitionDimension=1  PartitionWidth=1  PartitionOffset=0
  Source2 : Inport  Port=2  Partition=on  PartitionDimension=1  PartitionWidth=1  PartitionOffset=0
  Orientation : Inport  Port=3
  For Each : ForEach  DisableCoverage=on
  Orientation Swap : VectorOperationsLib/Orientation Swap
      settings: SourceProductName=Sydac Utilities
  WireState1 : Outport  ConcatenationDimension=1
  WireState2 : Outport  Port=2  ConcatenationDimension=1
  wires:
  Orientation/1 -> Orientation Swap/3
  Source2/1 -> Orientation Swap/2
  Orientation Swap/2 -> WireState2/1
  Orientation Swap/1 -> WireState1/1
  Source1/1 -> Orientation Swap/1

== system TCMSSystem/TCMSSystemPerVehicle/EnabledTCMSVehicle/TCMSDoors/DoorsDisplay/TCMSVehicleInfo/Subsystem1/For Each Subsystem4 ==
  Source1 : Inport  Partition=on  PartitionDimension=1  PartitionWidth=1  PartitionOffset=0
  Source2 : Inport  Port=2  Partition=on  PartitionDimension=1  PartitionWidth=1  PartitionOffset=0
  Orientation : Inport  Port=3
  For Each : ForEach  DisableCoverage=on
  Orientation Swap : VectorOperationsLib/Orientation Swap
      settings: SourceProductName=Sydac Utilities
  WireState1 : Outport  ConcatenationDimension=1
  WireState2 : Outport  Port=2  ConcatenationDimension=1
  wires:
  Source1/1 -> Orientation Swap/1
  Orientation Swap/1 -> WireState1/1
  Orientation Swap/2 -> WireState2/1
  Source2/1 -> Orientation Swap/2
  Orientation/1 -> Orientation Swap/3

== system TCMSSystem/TCMSSystemPerVehicle/EnabledTCMSVehicle/TCMSDoors/DoorsDisplay/TCMSVehicleInfo/Subsystem1/For Each Subsystem5 ==
  Source1 : Inport  Partition=on  PartitionDimension=1  PartitionWidth=1  PartitionOffset=0
  Source2 : Inport  Port=2  Partition=on  PartitionDimension=1  PartitionWidth=1  PartitionOffset=0
  Orientation : Inport  Port=3
  For Each : ForEach  DisableCoverage=on
  Orientation Swap : VectorOperationsLib/Orientation Swap
      settings: SourceProductName=Sydac Utilities
  WireState1 : Outport  ConcatenationDimension=1
  WireState2 : Outport  Port=2  ConcatenationDimension=1
  wires:
  Orientation/1 -> Orientation Swap/3
  Source2/1 -> Orientation Swap/2
  Orientation Swap/2 -> WireState2/1
  Orientation Swap/1 -> WireState1/1
  Source1/1 -> Orientation Swap/1

== system TCMSSystem/TCMSSystemPerVehicle/EnabledTCMSVehicle/TCMSDoors/DoorsDisplay/TCMSVehicleInfo/Subsystem1/For Each Subsystem6 ==
  Source1 : Inport  Partition=on  PartitionDimension=1  PartitionWidth=1  PartitionOffset=0
  Source2 : Inport  Port=2  Partition=on  PartitionDimension=1  PartitionWidth=1  PartitionOffset=0
  Orientation : Inport  Port=3
  For Each : ForEach  DisableCoverage=on
  Orientation Swap : VectorOperationsLib/Orientation Swap
      settings: SourceProductName=Sydac Utilities
  WireState1 : Outport  ConcatenationDimension=1
  WireState2 : Outport  Port=2  ConcatenationDimension=1
  wires:
  Source1/1 -> Orientation Swap/1
  Orientation Swap/1 -> WireState1/1
  Orientation Swap/2 -> WireState2/1
  Source2/1 -> Orientation Swap/2
  Orientation/1 -> Orientation Swap/3

== system TCMSSystem/TCMSSystemPerVehicle/EnabledTCMSVehicle/TCMSElectrical/ElectricalDisplay/EnableToRunScreen/CabUnitDisplay/CabActiveUnitDisplay ==
  In Bus Element1 : Inport  PortName=ElectricalSignals  Element=ForwardDirection
  In Bus Element2 : Inport  PortName=ElectricalSignals  Element=ReverseDirection
  In Bus Element5 : Inport  PortName=ElectricalSignals  Element=ParkBrakeApplication
  In Bus Element7 : Inport  PortName=ElectricalSignals  Element=NoLineVoltage
  In Bus Element8 : Inport  PortName=ElectricalSignals  Element=TractionSafe
  In Bus Element9 : Inport  PortName=ElectricalSignals  Element=DoorProvenLoopOK
  In Bus Element : Inport  PortName=ElectricalSignals  Element=MotorTrainLine
  In Bus Element4 : Inport  Port=2  PortName=WireStates  Element=PneumaticTrainSum.NoOfRPressCutout
  In Bus Element6 : Inport  Port=2  PortName=WireStates  Element=PneumaticTrainSum.NoOfEPICCutout
  In Bus Element11 : Inport  Port=2  PortName=WireStates  Element=PneumaticTrainSum.NoOfBrakesIsolated
  In Bus Element10 : Inport  Port=3  PortName=CBTC  Element=DriverModeSelection
  Action Port : ActionPort  ActionPortLabel=if(u1 > 0)
  Bus Creator : BusCreator  Inputs=14
  Constant{,7,12..13} (4 alike) : Constant  Value=0
  Data Type Conversion{,1..10} (11 alike) : DataTypeConversion
  Logical Operator1 : Logic  Operator=NOR  AllPortsSameDT=off  OutDataTypeStr=boolean
  Logical Operator2 : Logic  Operator=NOT  AllPortsSameDT=off  OutDataTypeStr=boolean
  Logical Operator3 : Logic  Operator=NOT  AllPortsSameDT=off  OutDataTypeStr=boolean
  Logical Operator4 : Logic  Operator=NOT  AllPortsSameDT=off  OutDataTypeStr=boolean
  More_Than_3_EPIC_Isolated : simulink/Logic and Bit Operations/Compare To Constant  relop=>  const=3  OutDataTypeStr=boolean
  More_Than_3_RPRESS_Isolated : simulink/Logic and Bit Operations/Compare To Constant  relop=>  const=3  OutDataTypeStr=boolean
  More_Than_6_Bogies_Isolated : simulink/Logic and Bit Operations/Compare To Constant  relop=>  const=6  OutDataTypeStr=boolean
  No_Mode : simulink/Logic and Bit Operations/Compare To Constant  relop===  const=0  OutDataTypeStr=boolean
  Out1 : Outport
  wires:
  Bus Creator/1 -> Out1/1
  Data Type Conversion6/1 -> Bus Creator/13  "ParkBrakeApplied"
  In Bus Element9/1 -> Logical Operator2/1
  In Bus Element2/1 -> Logical Operator1/2
  Data Type Conversion9/1 -> Bus Creator/3  "NoModeSelected"
  Data Type Conversion4/1 -> Bus Creator/2  "NoCabActive"
  Data Type Conversion7/1 -> Bus Creator/12  "BrakeLoopCutout"
  Logical Operator2/1 -> Data Type Conversion8/1
  No_Mode/1 -> Data Type Conversion9/1
  Data Type Conversion8/1 -> Bus Creator/14  "DoorLoopNotOK"
  In Bus Element5/1 -> Data Type Conversion6/1
  Data Type Conversion3/1 -> Bus Creator/4  "NoDirectionSelected"
  Data Type Conversion2/1 -> Bus Creator/7  "TooManyRPRESS"
  In Bus Element1/1 -> Logical Operator1/1
  Data Type Conversion/1 -> Bus Creator/9  "TooManyBogies"
  Data Type Conversion5/1 -> Bus Creator/1  "NoLineVoltage"
  Logical Operator1/1 -> Data Type Conversion3/1
  More_Than_3_RPRESS_Isolated/1 -> Data Type Conversion2/1
  More_Than_3_EPIC_Isolated/1 -> Data Type Conversion1/1
  Data Type Conversion1/1 -> Bus Creator/8  "TooManyEPIC"
  In Bus Element6/1 -> More_Than_3_EPIC_Isolated/1
  In Bus Element11/1 -> More_Than_6_Bogies_Isolated/1
  More_Than_6_Bogies_Isolated/1 -> Data Type Conversion/1
  In Bus Element8/1 -> Logical Operator3/1
  In Bus Element7/1 -> Data Type Conversion5/1
  Constant/1 -> Data Type Conversion4/1
  In Bus Element4/1 -> More_Than_3_RPRESS_Isolated/1
  In Bus Element10/1 -> No_Mode/1
  Constant12/1 -> Bus Creator/6  "TrainReadyNotOK"
  Constant7/1 -> Bus Creator/5  "ATCStatusNotOK"
  Data Type Conversion10/1 -> Bus Creator/11  "MotoringTLDeenergized"
  Constant13/1 -> Bus Creator/10  "ZVRDNotActive"
  Logical Operator3/1 -> Data Type Conversion7/1
  In Bus Element/1 -> Logical Operator4/1
  Logical Operator4/1 -> Data Type Conversion10/1

== system TCMSSystem/TCMSSystemPerVehicle/EnabledTCMSVehicle/TCMSElectrical/ElectricalDisplay/EnableToRunScreen/CabUnitDisplay/CabInActiveUnitDisplay ==
  Action Port : ActionPort  ActionPortLabel=else
  Bus Creator : BusCreator  Inputs=14
  Constant{,2..13} (13 alike) : Constant  Value=0
  Constant1 : Constant
  Out1 : Outport
  wires:
  Constant1/1 -> Bus Creator/2  "NoCabActive"
  Constant/1 -> Bus Creator/1  "NoLineVoltage"
  Bus Creator/1 -> Out1/1
  Constant7/1 -> Bus Creator/5  "ATCStatusNotOK"
  Constant4/1 -> Bus Creator/7  "TooManyRPRESS"
  Constant9/1 -> Bus Creator/13  "ParkBrakeApplied"
  Constant8/1 -> Bus Creator/12  "BrakeLoopCutout"
  Constant5/1 -> Bus Creator/8  "TooManyEPIC"
  Constant10/1 -> Bus Creator/14  "DoorLoopNotOK"
  Constant3/1 -> Bus Creator/4  "NoDirectionSelected"
  Constant6/1 -> Bus Creator/9  "TooManyBogies"
  Constant2/1 -> Bus Creator/3  "NoModeSelected"
  Constant12/1 -> Bus Creator/6  "TrainReadyNotOK"
  Constant13/1 -> Bus Creator/10  "ZVRDNotActive"
  Constant11/1 -> Bus Creator/11  "MotoringTLDeenergized"

== system TCMSSystem/TCMSSystemPerVehicle/EnabledTCMSVehicle/TCMSElectrical/ElectricalDisplay/OperatingandHeaderScreen/CabUnitDisplay/CabActiveUnitDisplay ==
  In Bus Element4 : Inport  PortName=ElectricalSignals  Element=CabActive
  In Bus Element : Inport  PortName=ElectricalSignals  Element=HMIPower
  Action Port : ActionPort  ActionPortLabel=if(u1 > 0)
  Bus Creator : BusCreator  Inputs=2
  Data Type Conversion : DataTypeConversion  OutDataTypeStr=double
  Data Type Conversion1 : DataTypeConversion  OutDataTypeStr=double
  Out1 : Outport
  wires:
  Data Type Conversion1/1 -> Bus Creator/2  "CabActive"
  Data Type Conversion/1 -> Bus Creator/1  "HMIPower"
  In Bus Element4/1 -> Data Type Conversion1/1
  In Bus Element/1 -> Data Type Conversion/1
  Bus Creator/1 -> Out1/1

== system TCMSSystem/TCMSSystemPerVehicle/EnabledTCMSVehicle/TCMSElectrical/ElectricalDisplay/OperatingandHeaderScreen/CabUnitDisplay/CabInActiveUnitDisplay ==
  Action Port : ActionPort  ActionPortLabel=else
  Bus Creator : BusCreator  Inputs=2
  Constant : Constant  Value=0
  Constant1 : Constant  Value=0
  Out1 : Outport
  wires:
  Constant1/1 -> Bus Creator/2  "CabActive"
  Constant/1 -> Bus Creator/1  "HMIPower"
  Bus Creator/1 -> Out1/1

== system TCMSSystem/TCMSSystemPerVehicle/EnabledTCMSVehicle/TCMSElectrical/ElectricalDisplay/OperatingandHeaderScreen/Subsystem/If Action Subsystem ==
  Action Port : ActionPort  ActionPortLabel=if(u1 & ~u3)
  Constant : Constant  Value=3
  Out1 : Outport
  wires:
  Constant/1 -> Out1/1

== system TCMSSystem/TCMSSystemPerVehicle/EnabledTCMSVehicle/TCMSElectrical/ElectricalDisplay/OperatingandHeaderScreen/Subsystem/If Action Subsystem1 ==
  Action Port : ActionPort  ActionPortLabel=elseif(u1 & u3)
  Constant : Constant  Value=9
  Out1 : Outport
  wires:
  Constant/1 -> Out1/1

== system TCMSSystem/TCMSSystemPerVehicle/EnabledTCMSVehicle/TCMSElectrical/ElectricalDisplay/OperatingandHeaderScreen/Subsystem/If Action Subsystem2 ==
  Action Port : ActionPort  ActionPortLabel=elseif( ~u1 & (u2 | u3) )
  Constant : Constant  Value=8
  Out1 : Outport
  wires:
  Constant/1 -> Out1/1

== system TCMSSystem/TCMSSystemPerVehicle/EnabledTCMSVehicle/TCMSTractionBraking/TractionBrakingControl/CabControlsExtract/Speed Limit Protection/0kphConditions ==
  note: Conditions for 0 Kph
      | Direction Switch at Standby/Off
  PneumaticTrainSum : Inport
  IOControls : Inport  Port=2
  CBTCIn : Inport  Port=3
  AND : Logic  AllPortsSameDT=off  OutDataTypeStr=boolean
  AND1 : Logic  Operator=OR  Inputs=3  AllPortsSameDT=off  OutDataTypeStr=boolean
  AND2 : Logic  Operator=OR  AllPortsSameDT=off  OutDataTypeStr=boolean
  ATO : simulink/Logic and Bit Operations/Compare To Constant  relop===  const=5  OutDataTypeStr=boolean
  ATP : simulink/Logic and Bit Operations/Compare To Constant  relop===  const=4  OutDataTypeStr=boolean
  Bus Selector1 : BusSelector  OutputSignals=NoOfBogieIsolated
  Bus Selector2 : BusSelector  OutputSignals=ModeSelector
  Bus Selector3 : BusSelector  OutputSignals=ATCBypassState
  More_Than_6_Bogies_Isolated : simulink/Logic and Bit Operations/Compare To Constant  relop=>  const=6  OutDataTypeStr=boolean
  UTO : simulink/Logic and Bit Operations/Compare To Constant  relop===  const=0  OutDataTypeStr=boolean
  True : Outport
  wires:
  PneumaticTrainSum/1 -> Bus Selector1/1
  Bus Selector1/1 -> More_Than_6_Bogies_Isolated/1  "<NoOfBogieIsolated>"
  More_Than_6_Bogies_Isolated/1 -> AND1/1  "ZeroLimit"
  ATP/1 -> AND2/1
  Bus Selector2/1 -> UTO/1, ATO/1, ATP/1  "<ModeSelector>"
  Bus Selector3/1 -> AND/1  "<ATCBypassState>"
  CBTCIn/1 -> Bus Selector3/1
  IOControls/1 -> Bus Selector2/1
  AND1/1 -> True/1
  AND/1 -> AND1/2
  AND2/1 -> AND/2
  ATO/1 -> AND2/2
  UTO/1 -> AND1/3

== system TCMSSystem/TCMSSystemPerVehicle/EnabledTCMSVehicle/TCMSTractionBraking/TractionBrakingControl/CabControlsExtract/Speed Limit Protection/10kphConditions ==
  note: Conditions for 10 Kph
      | Restricted Reverse Mode
  PneumaticsIn : Inport
  CBTCIn : Inport  Port=2
  IOControls : Inport  Port=3
  AND : Logic  AllPortsSameDT=off  OutDataTypeStr=boolean
  Bus Selector1 : BusSelector  OutputSignals=ATCBypassState
  Bus Selector2 : BusSelector  OutputSignals=NoOfBogieIsolated
  Bus Selector3 : BusSelector  OutputSignals=ModeSelector
  Exactly_6_Bogies_Isolated : simulink/Logic and Bit Operations/Compare To Constant  relop===  const=6  OutDataTypeStr=boolean
  OR2 : Logic  Operator=OR  AllPortsSameDT=off  OutDataTypeStr=boolean
  RMR : simulink/Logic and Bit Operations/Compare To Constant  relop===  const=1  OutDataTypeStr=boolean
  True : Outport
  wires:
  PneumaticsIn/1 -> Bus Selector2/1
  Bus Selector2/1 -> Exactly_6_Bogies_Isolated/1  "<NoOfBogieIsolated>"
  Exactly_6_Bogies_Isolated/1 -> OR2/1
  CBTCIn/1 -> Bus Selector1/1
  IOControls/1 -> Bus Selector3/1
  Bus Selector3/1 -> RMR/1  "<ModeSelector>"
  RMR/1 -> AND/2
  AND/1 -> OR2/2
  OR2/1 -> True/1  "Restricted"
  Bus Selector1/1 -> AND/1  "<ATCBypassState>"

== system TCMSSystem/TCMSSystemPerVehicle/EnabledTCMSVehicle/TCMSTractionBraking/TractionBrakingControl/CabControlsExtract/Speed Limit Protection/25kphConditions ==
  note: Conditions for 25 Kph
      | Safety Cutout/ATC bypass mode
      | Restricted Forward Mode
      | Limp Home Mode
  IOControls : Inport
  CBTCIn : Inport  Port=2
  ElectricalIn : Inport  Port=3
  AND : Logic  AllPortsSameDT=off  OutDataTypeStr=boolean
  Bus Selector1 : BusSelector  OutputSignals=ModeSelector
  Bus Selector2 : BusSelector  OutputSignals=ATCBypassState
  Bus Selector3 : BusSelector  OutputSignals=LimpHomeMode
  OR2 : Logic  Operator=OR  AllPortsSameDT=off  OutDataTypeStr=boolean
  RMF : simulink/Logic and Bit Operations/Compare To Constant  relop===  const=3  OutDataTypeStr=boolean
  True : Outport
  wires:
  CBTCIn/1 -> Bus Selector2/1
  OR2/1 -> True/1  "Restricted"
  Bus Selector3/1 -> OR2/2  "<LimpHomeMode>"
  ElectricalIn/1 -> Bus Selector3/1
  Bus Selector1/1 -> RMF/1  "<ModeSelector>"
  IOControls/1 -> Bus Selector1/1
  Bus Selector2/1 -> AND/2  "<ATCBypassState>"
  RMF/1 -> AND/1
  AND/1 -> OR2/1

== system TCMSSystem/TCMSSystemPerVehicle/EnabledTCMSVehicle/TCMSTractionBraking/TractionBrakingControl/CabControlsExtract/Speed Limit Protection/40kphConditions ==
  note: Conditions for 40 Kph
      |
      | 4 bogies isolated due to any of the isolation cocks
  ElectricalIn : Inport
  PneumaticTrainSum : Inport  Port=2
  TractionBrakingBogieData : Inport  Port=3
  <Bogie> : Inport  Port=4
  6_Bogies_Isolated : simulink/Logic and Bit Operations/Compare To Constant  relop=>=  const=4  OutDataTypeStr=boolean
  Bus Selector1 : BusSelector  OutputSignals=NoOfBogieIsolated
  Bus Selector2 : BusSelector  OutputSignals=Speedometer
  For Each Subsystem : Subsystem  TreatAsAtomicUnit=on
  Logical Operator : Logic  Operator=OR  Inputs=1  AllPortsSameDT=off  OutDataTypeStr=boolean
  Logical Operator2 : Logic  Operator=OR  Inputs=3  AllPortsSameDT=off  OutDataTypeStr=boolean
  Logical Operator3 : Logic  Operator=OR  Inputs=1  AllPortsSameDT=off  OutDataTypeStr=boolean
  OR2 : Logic  Operator=OR  Inputs=1  AllPortsSameDT=off  OutDataTypeStr=boolean
  Subsystem : Subsystem
  True : Outport
  wires:
  6_Bogies_Isolated/1 -> Logical Operator/1
  Bus Selector1/1 -> 6_Bogies_Isolated/1  "<NoOfBogieIsolated>"
  PneumaticTrainSum/1 -> Bus Selector1/1
  Logical Operator/1 -> Logical Operator2/1
  TractionBrakingBogieData/1 -> For Each Subsystem/1(In1)
  Logical Operator2/1 -> True/1
  Subsystem/1(<BECU1LoadPressureLow>) -> OR2/1
  <Bogie>/1 -> Subsystem/1(In1)
  OR2/1 -> Logical Operator2/3
  For Each Subsystem/1(Out2) -> Logical Operator3/1
  Logical Operator3/1 -> Logical Operator2/2
  ElectricalIn/1 -> Bus Selector2/1
  Bus Selector2/1 -> For Each Subsystem/2(Speedometer)  "<Speedometer>"

== system TCMSSystem/TCMSSystemPerVehicle/EnabledTCMSVehicle/TCMSTractionBraking/TractionBrakingControl/CabControlsExtract/Speed Limit Protection/45kphConditions ==
  note: Conditions for 45 Kph
      | 3 bogies isolated due to any of the isolation cocks
  PneumaticTrainSum : Inport
  3_Bogies_Isolated : simulink/Logic and Bit Operations/Compare To Constant  relop=>=  const=3  OutDataTypeStr=boolean
  Bus Selector1 : BusSelector  OutputSignals=NoOfBogieIsolated
  OR1 : Logic  Operator=OR  Inputs=1  AllPortsSameDT=off  OutDataTypeStr=boolean
  True : Outport
  wires:
  PneumaticTrainSum/1 -> Bus Selector1/1
  Bus Selector1/1 -> 3_Bogies_Isolated/1  "<NoOfBogieIsolated>"
  3_Bogies_Isolated/1 -> OR1/1
  OR1/1 -> True/1  "NoDirection"
